simulink model "MySusp_Damper_RTW"  (Simulink 10.3)
settings: Solver=ode1  StartTime=0.0  StopTime=inf  FixedStep=0.001  RelTol=1e-3
PreLoadFcn:
  | vehicle = 'Car'; if ~length(which('cmself')), cmenv; end
  | MySusp_Damper_RTW_bus
  | MySusp_Damper_RTW_params
InitFcn:
  | vehicle = 'Car'; if ~length(which('cmself')), cmenv; end
  | MySusp_Damper_RTW_bus
undefined symbols (not defined in the file or in its folder): Damping_Pull, Damping_Push
Description:
  | CarMaker Plug-in Model Target
settings Model: Creator=ml  ModifiedByFormat=IPG  LastModifiedBy=IPG  MultithreadedSim=on
settings DataIOCC: SaveFormat=Dataset  SignalLoggingSaveFormat=Dataset
settings OptimizationCC: ExpressionDepthLimit=128  LifeSpan=auto
settings DebuggingCC: UnderspecifiedInitializationDetection=Simplified  MergeDetectMultiDrivingBlocksExec=error  FcnCallInpInsideContextMsg=error  StateNameClashWarn=none  PregeneratedLibrarySubsystemCodeDiagnostic=none  SFUnexpectedBacktrackingDiag=error  SFNoUnconditionalDefaultTransitionDiag=error  SFExecutionAtInitializationDiag=warning
settings HardwareCC: ProdBitPerPointer=64  ProdBitPerSizeT=64  ProdBitPerPtrDiffT=64  ProdLargestAtomicFloat=Float  ProdIntDivRoundTo=Zero  ProdEndianess=LittleEndian  ProdWordSize=64  ProdHWDeviceType=Intel->x86-64 (Windows64)
settings ModelReferenceCC: PropagateSignalLabelsOutOfModel=on
settings RTWCC: Description=CarMaker Plug-in Model Target  SystemTargetFile=CarMaker.tlc  TemplateMakefile=CarMaker_unix-win64.tmf
settings CodeAppCC: MaxIdLength=127
settings STFCustomTargetCC: TargetLangStandard=C99 (ISO)  CombineOutputUpdateFcns=on  CodeInterfacePackaging=Reusable function  GRTInterface=off  GenerateAllocFcn=on  SystemTargetFile=CarMaker.tlc
settings GRTTargetCC: TargetLangStandard=C99 (ISO)  ParMdlRefBuildCompliant=off  CompOptLevelCompliant=off  ConcurrentExecutionCompliant=off  CombineOutputUpdateFcns=on  MatFileLogging=off  CodeInterfacePackaging=Reusable function  CPPClassGenCompliant=off  GRTInterface=off  GenerateAllocFcn=on  UseToolchainInfoCompliant=off  RTWCAPISignals=on  RTWCAPIParams=on  RTWCAPIStates=on
settings CustomProperty: DataType=string
settings EnumStrPairs: String=Car
settings ConfigComp: CovMetricSettings=dwe  CovSaveCumulativeToWorkspaceVar=off  CovSaveSingleToWorkspaceVar=off  CovExternalEMLEnable=on

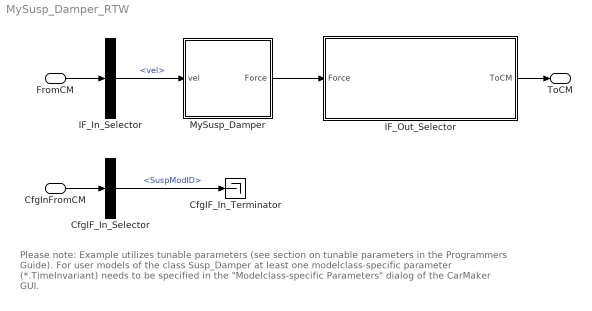
== system MySusp_Damper_RTW ==
  note: Please note: Example utilizes tunable parameters (see section on tunable parameters in the Programmers Guide).
      |
      | For user models of the class Susp_Damper at least one modelclass-specific parameter (*.TimeInvariant) needs to be specified in the
      | "Modelclass-specific Parameters" dialog of the CarMaker GUI.
  FromCM : Inport  OutDataTypeStr=Bus: cmSusp_DamperIn
  CfgInFromCM : Inport  Port=2  OutDataTypeStr=Bus: cmSusp_DamperCfgIn
  CfgIF_In_Selector : BusSelector  OutputSignals=SuspModID
  CfgIF_In_Terminator : Terminator
  IF_In_Selector : BusSelector  OutputSignals=vel
  IF_Out_Selector : Subsystem  mask(Signal Selection){}
      mask help: Signal Selection Block
      settings: OpenFcn=cmSignalSelect('SignalSelection_CB',gcb)
  MySusp_Damper : Subsystem
  ToCM : Outport  OutDataTypeStr=Bus: cmSusp_DamperOut  VectorParamsAs1DForOutWhenUnconnected=off
  wires:
  FromCM/1 -> IF_In_Selector/1
  IF_Out_Selector/1(ToCM) -> ToCM/1
  CfgInFromCM/1 -> CfgIF_In_Selector/1
  CfgIF_In_Selector/1 -> CfgIF_In_Terminator/1  "<SuspModID>"
  IF_In_Selector/1 -> MySusp_Damper/1(vel)  "<vel>"
  MySusp_Damper/1(Force) -> IF_Out_Selector/1(Force)

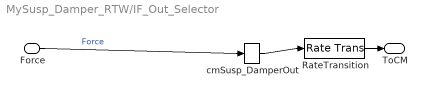
== system MySusp_Damper_RTW/IF_Out_Selector ==
  Force : Inport
  RateTransition : RateTransition  OutPortSampleTime=str2num(get_param(bdroot,'FixedStep'))
  cmSusp_DamperOut : BusCreator  Inputs=1
  ToCM : Outport  VectorParamsAs1DForOutWhenUnconnected=off
  wires:
  RateTransition/1 -> ToCM/1
  cmSusp_DamperOut/1 -> RateTransition/1
  Force/1 -> cmSusp_DamperOut/1  "Force"

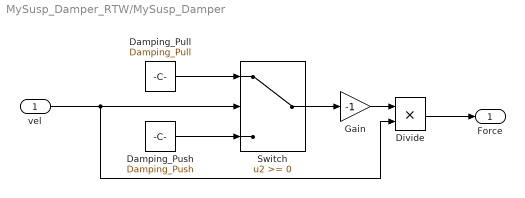
== system MySusp_Damper_RTW/MySusp_Damper ==
  vel : Inport
  Damping_Pull : Constant  Value=Damping_Pull
  Damping_Push : Constant  Value=Damping_Push
  Divide : Product  Inputs=**
  Gain : Gain  Gain=-1
  Switch : Switch
  Force : Outport  VectorParamsAs1DForOutWhenUnconnected=off
  wires:
  vel/1 -> Divide/2, Switch/2
  Switch/1 -> Gain/1
  Damping_Pull/1 -> Switch/1
  Damping_Push/1 -> Switch/3
  Gain/1 -> Divide/1
  Divide/1 -> Force/1
